simulink model "case_3_lead_rapid_increase_space"  (R2025b)
settings: Solver=VariableStepAuto  StartTime=0.0  StopTime=10.0  RelTol=1e-3
settings Model: Creator=sanborkl  LastModifiedBy=admin

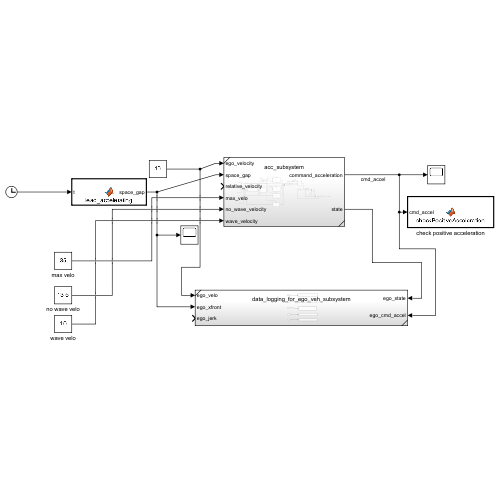
[thumbnail: Simulink's stored preview of the top-level diagram]
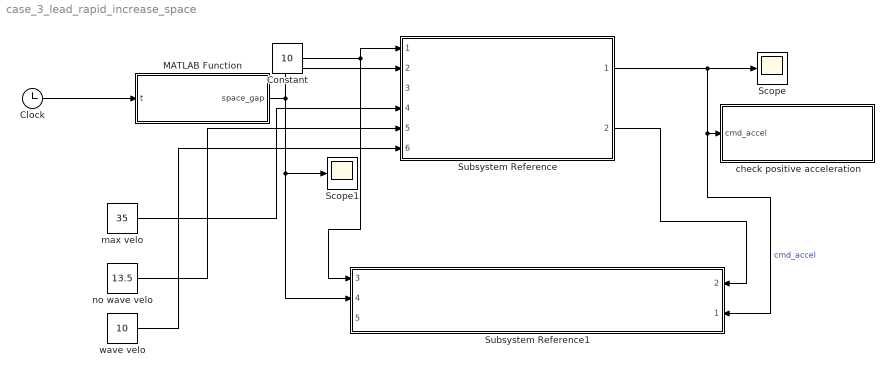
== system case_3_lead_rapid_increase_space ==
  Clock : Clock
  Constant : Constant  Value=10
  MATLAB Function : MATLAB Function  TreatAsAtomicUnit=on
  Scope : Scope
      settings: ActiveDisplayYMinimum=-2.8888932305545127  ActiveDisplayYMaximum=0.71887853146030856
  Scope1 : Scope
      settings: ActiveDisplayYMinimum=13.750000000000002  ActiveDisplayYMaximum=76.25
  Subsystem Reference : Subsystem  ReferencedSubsystem=acc_subsystem
  Subsystem Reference1 : Subsystem  ReferencedSubsystem=data_logging_for_ego_veh_subsystem
      settings: PortSchema="{\"entries\":[{\"content\":{\"sides\":[{\"content\":{\"connectorIds\":[\"In3\",\"In4\",\"In5\"]},\"type\":\"ConnectorPlacement.EquallySpacedRectSide\",\"uuid\":\"0b96bcaa-a470-46c9-9268-f4bd6b1035a8\"},{\"content\":{\"connectorIds\":[\"In2\",\"In1\"],\"side\":\"RIGHT\"},\"type\":\"ConnectorPlacement.EquallySpacedRectSide\",\"uuid\":\"8e49005a-1e53-4e76-b163-50df0eb9f2cc\"},{\"content\":{\"side\":\"TOP\"},\"type\":\"ConnectorPlacement.EquallySpacedRectSide\",\"uuid\":\"3ff4af65-efca-4a64-9b7f-f479498e89e2\"}]},\"type\":\"ConnectorPlacement.EquallySpacedConnector\",\"uuid\":\"f10caef7-9599-4d5c-a8fd-3eb49f6fcaa8\"}],\"packageUris\":[\"http://schema.mathworks.com/mf0/Connector/R2020b\"],\"version\":\"1.0\"}"
  check positive acceleration : MATLAB Function  TreatAsAtomicUnit=on
  max velo : Constant  Value=35
  no wave velo : Constant  Value=13.5
  wave velo : Constant  Value=10
  wires:
  MATLAB Function/1(space_gap) -> Subsystem Reference1/4, Scope1/1, Subsystem Reference/2
  Clock/1 -> MATLAB Function/1(t)
  Subsystem Reference/1 -> Subsystem Reference1/1, check positive acceleration/1(cmd_accel), Scope/1  "cmd_accel"
  Constant/1 -> Subsystem Reference1/3, Subsystem Reference/1
  Subsystem Reference/2 -> Subsystem Reference1/2
  max velo/1 -> Subsystem Reference/4
  no wave velo/1 -> Subsystem Reference/5
  wave velo/1 -> Subsystem Reference/6

== matlab function case_3_lead_rapid_increase_space/check positive acceleration ==
  data: cmd_accel input
function checkPositiveAcceleration(cmd_accel)
%#codegen
coder.extrinsic('disp', 'sprintf');

if cmd_accel < 0
    msg = sprintf('Error: Negative command acceleration: %.3f, should be positive', ...
                  cmd_accel);
    disp(msg);
end
end

== matlab function case_3_lead_rapid_increase_space/MATLAB Function ==
  data: t input; space_gap output
function space_gap = lead_accelerating(t)

space_gap = 35 + 5 * t;
